simulink model "A6_S36_Totzeit"  (R2015a)
settings: Solver=ode45  StartTime=0.0  StopTime=500  RelTol=1e-3
settings Model: Creator=James  LastModifiedBy=James

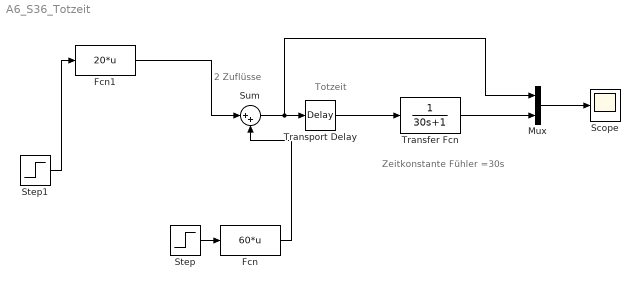
== system A6_S36_Totzeit ==
  note: Zeitkonstante Fühler =30s
  note: Totzeit
  note: 2 Zuflüsse
  Fcn : Fcn  Expr=60*u
  Fcn1 : Fcn  Expr=20*u
  Mux : Mux  Inputs=2
  Scope : Scope
  Step : Step  Time=200  After=0.5  SampleTime=0
  Step1 : Step  Time=200  Before=1  After=0.5  SampleTime=0
  Sum : Sum  Inputs=|++
  Transfer Fcn : TransferFcn  Denominator=[30 1]
  Transport Delay : TransportDelay  DelayTime=10
  wires:
  Step1/1 -> Fcn1/1
  Step/1 -> Fcn/1
  Sum/1 -> Mux/1, Transport Delay/1
  Transport Delay/1 -> Transfer Fcn/1
  Transfer Fcn/1 -> Mux/2
  Mux/1 -> Scope/1
  Fcn1/1 -> Sum/1
  Fcn/1 -> Sum/2
